simulink model "wlan_mac_dcf_hw"  (Simulink 7.7)
settings: Solver=ode45  StartTime=0.0  StopTime=2e4  RelTol=1e-3
PostLoadFcn:
  | wlan_mac_hw_init
InitFcn:
  | wlan_mac_hw_init
StartFcn:
  | wlan_mac_hw_init
values from neighbouring files (symbols this model uses):
  NB_CNTR_NAV = ceil(log2(MAX_NAV * 160))    [wlan_mac_hw_init.m]
  ticks_per_usec = 10    [wlan_mac_hw_init.m]
undefined symbols (not defined in the file or in its folder): gcbh, xlBlockLoadCallback, xlGetNormalizedPeriod
libraries: xbsIndex_r4 x552, xbsEDKLib_r4 x1
(part 3 of 5)

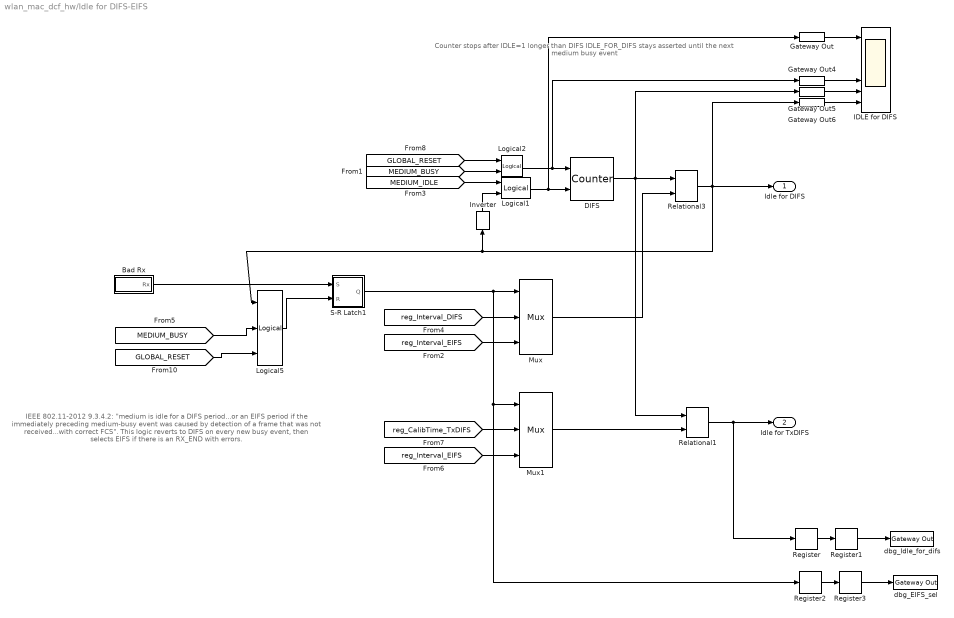
== system wlan_mac_dcf_hw/Idle for DIFS-EIFS ==
  note: IEEE 802.11-2012 9.3.4.2:
      | "medium is idle for a DIFS period...or an EIFS period if the immediately preceding medium-busy
      | event was caused by detection of a frame that was not received...with correct FCS".
      |
      | This logic reverts to DIFS on every new busy event, then
      | selects EIFS if there is an RX_END with errors.
  note: Counter stops after IDLE=1 longer than DIFS
      | IDLE_FOR_DIFS stays asserted until
      | the next medium busy event
  Bad Rx : Subsystem
  DIFS : xbsIndex_r4/Counter  cnt_type=Free Running  cnt_to=inf  operation=Up  start_count=0  cnt_by_val=1  arith_type=Unsigned  n_bits=NB_CNTR_DIFS  bin_pt=0  load_pin=off  rst=on  en=on  explicit_period=off  period=1  dbl_ovrd=off  use_behavioral_HDL=off  implementation=Fabric  block_type=counter
  Gateway Out{,4..6} (4 alike) : xbsIndex_r4/Gateway Out  inherit_from_input=off  hdl_port=off  timing_constraint=None  locs_specified=off  LOCs={}  UseAsDAC=off  DACChannel='1'  block_type=gatewayout
  IDLE for DIFS : Scope  NumInputPorts=7
      settings: YMin=-5~-5~-5~-5~-5~-5~-5  YMax=5~5~5~5~5~5~5  SaveName=ScopeData4
  Inverter : xbsIndex_r4/Inverter  en=off  latency=0  dbl_ovrd=off  block_type=inv
      settings: xl_area=[0 0 0 0 0 0 0]  block_version=VER_STRING_GOES_HERE
  Logical1 : xbsIndex_r4/Logical  logical_function=AND  inputs=2  en=off  latency=0  precision=Full  arith_type=Unsigned  n_bits=16  bin_pt=0  align_bp=on  dbl_ovrd=off  block_type=logical
  Logical2 : xbsIndex_r4/Logical  logical_function=OR  inputs=2  en=off  latency=0  precision=Full  arith_type=Unsigned  n_bits=8  bin_pt=2  align_bp=on  dbl_ovrd=off  block_type=logical
      settings: xl_area=[1 0 0 1 0 0 0]  block_version=VER_STRING_GOES_HERE
  Logical5 : xbsIndex_r4/Logical  logical_function=OR  inputs=3  en=off  latency=0  precision=Full  arith_type=Unsigned  n_bits=16  bin_pt=0  align_bp=on  dbl_ovrd=off  block_type=logical
  Mux : xbsIndex_r4/Mux  inputs=2  en=off  latency=0  precision=Full  arith_type=Unsigned  n_bits=16  bin_pt=14  quantization=Truncate  overflow=Wrap  dbl_ovrd=off  block_type=mux
  Mux1 : xbsIndex_r4/Mux  inputs=2  en=off  latency=0  precision=Full  arith_type=Unsigned  n_bits=16  bin_pt=14  quantization=Truncate  overflow=Wrap  dbl_ovrd=off  block_type=mux
  Register{,1..3} (4 alike) : xbsIndex_r4/Register  init=0  rst=off  en=off  dbl_ovrd=off  block_type=register
  Relational1 : xbsIndex_r4/Relational  mode=a>=b  en=off  latency=0  dbl_ovrd=off  block_type=relational
  Relational3 : xbsIndex_r4/Relational  mode=a>=b  en=off  latency=0  dbl_ovrd=off  block_type=relational
  S-R Latch1 : Subsystem
  dbg_EIFS_sel : xbsIndex_r4/Gateway Out  inherit_from_input=off  hdl_port=on  timing_constraint=None  locs_specified=off  LOCs={}  UseAsDAC=off  DACChannel='1'  block_type=gatewayout
  dbg_Idle_for_difs : xbsIndex_r4/Gateway Out  inherit_from_input=off  hdl_port=on  timing_constraint=None  locs_specified=off  LOCs={}  UseAsDAC=off  DACChannel='1'  block_type=gatewayout
  Idle for DIFS : Outport
  Idle for TxDIFS : Outport  Port=2
  wires:
  Relational3/1 -> Idle for DIFS/1, Inverter/1, Logical5/1, Gateway Out6/1
  Mux/1 -> Relational3/2
  DIFS/1 -> Relational3/1, Relational1/1, Gateway Out5/1
  Logical2/1 -> DIFS/1, Gateway Out4/1
  Logical1/1 -> DIFS/2, Gateway Out/1
  [MEDIUM_IDLE] -> Logical1/1
  [reg_Interval_DIFS] -> Mux/2
  [reg_Interval_EIFS] -> Mux/3
  S-R Latch1/1(Q) -> Mux/1, Mux1/1, Register2/1
  Bad Rx/1(Rx) -> S-R Latch1/1(S)
  Logical5/1 -> S-R Latch1/2(R)
  [MEDIUM_BUSY] -> Logical5/2
  [reg_CalibTime_TxDIFS] -> Mux1/2
  [reg_Interval_EIFS] -> Mux1/3
  Mux1/1 -> Relational1/2
  Relational1/1 -> Idle for TxDIFS/1, Register/1
  Inverter/1 -> Logical1/2
  Gateway Out/1 -> IDLE for DIFS/1
  Gateway Out4/1 -> IDLE for DIFS/5
  Gateway Out5/1 -> IDLE for DIFS/6
  Gateway Out6/1 -> IDLE for DIFS/7
  [GLOBAL_RESET] -> Logical5/3
  [MEDIUM_BUSY] -> Logical2/2
  [GLOBAL_RESET] -> Logical2/1
  Register/1 -> Register1/1
  Register1/1 -> dbg_Idle_for_difs/1
  Register2/1 -> Register3/1
  Register3/1 -> dbg_EIFS_sel/1

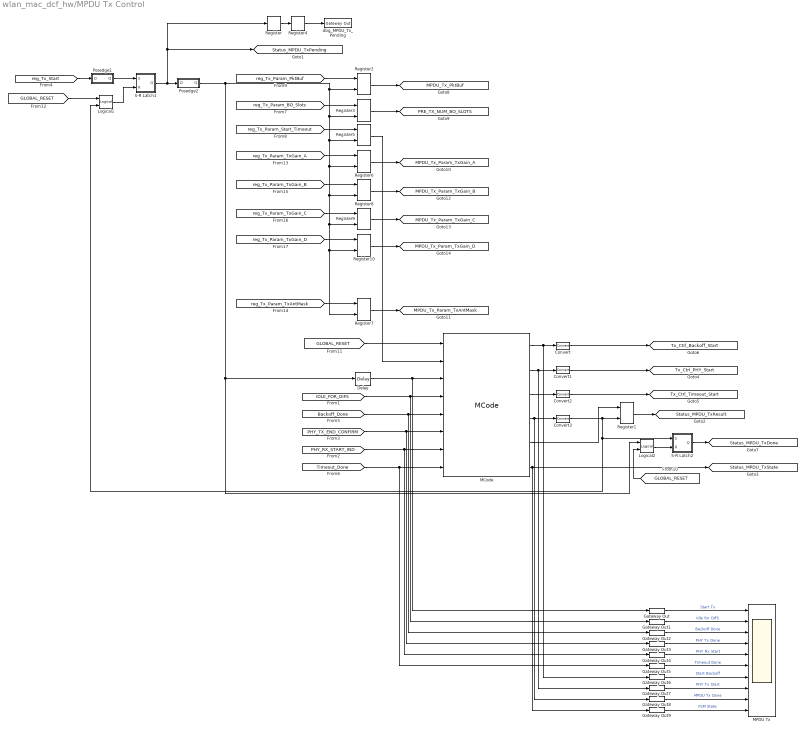
== system wlan_mac_dcf_hw/MPDU Tx Control ==
  Convert{,1..3} (4 alike) : xbsIndex_r4/Convert  gui_display_data_type=Boolean  arith_type=Boolean  n_bits=16  bin_pt=14  float_type=Single  exp_bits=8  fraction_bits=24  quantization=Truncate  overflow=Wrap  en=off  latency=0  dbl_ovrd=off  pipeline=off  block_type=convert
  Delay : xbsIndex_r4/Delay  rst=off  infoeditControl=Selection of Reset will increase slice count due to use of real FFs and instead of SRLs  en=off  latency=1  dbl_ovrd=off  reg_retiming=off  block_type=delay
  Gateway Out{,1..9} (10 alike) : xbsIndex_r4/Gateway Out  inherit_from_input=off  hdl_port=off  timing_constraint=None  locs_specified=off  LOCs={}  UseAsDAC=off  DACChannel='1'  block_type=gatewayout
  Logical1 : xbsIndex_r4/Logical  logical_function=OR  inputs=2  en=off  latency=0  precision=Full  arith_type=Unsigned  n_bits=8  bin_pt=2  align_bp=on  dbl_ovrd=off  block_type=logical
      settings: xl_area=[1 0 0 1 0 0 0]  block_version=VER_STRING_GOES_HERE
  Logical2 : xbsIndex_r4/Logical  logical_function=OR  inputs=2  en=off  latency=0  precision=Full  arith_type=Unsigned  n_bits=8  bin_pt=2  align_bp=on  dbl_ovrd=off  block_type=logical
      settings: xl_area=[1 0 0 1 0 0 0]  block_version=VER_STRING_GOES_HERE
  MCode : xbsIndex_r4/MCode  mfname=mac_tx_ctrl_fsm  explicit_period=on  period=1  inputsTable={'boundInpExpr'=>['','','','','','','',''],'inputs'=>['reset','timeout_req','new_tx','idle_for_difs','backoff_done','phy_tx_done','phy_rx_start','timeout_done']}  outputsTable={'outputs'=>['backoff_start','phy_tx_start','timeout_start','tx_done','tx_result_out','fsm_state_out'],'suppressOut'=>['off','off','off','off','off','off']}  dbl_ovrd=off  enable_stdout=off  enable_debug=off  suppress_output=on  defparams={}  hide_port_list={}  block_type=mcode
  MPDU Tx : Scope  NumInputPorts=10
      settings: YMin=-5~-5~-5~-5~-5~-5~-5~-5~-5~-5  YMax=5~5~5~5~5~5~5~5~5~5
  Posedge1 : Subsystem
  Posedge2 : Subsystem
  Register : xbsIndex_r4/Register  init=0  rst=off  en=off  dbl_ovrd=off  block_type=register
  Register{1..3,5..10} (9 alike) : xbsIndex_r4/Register  init=0  rst=off  en=on  dbl_ovrd=off  block_type=register
  Register4 : xbsIndex_r4/Register  init=0  rst=off  en=off  dbl_ovrd=off  block_type=register
  S-R Latch1 : Subsystem
  S-R Latch2 : Subsystem
  dbg_MPDU_Tx_Pending : xbsIndex_r4/Gateway Out  inherit_from_input=off  hdl_port=on  timing_constraint=None  locs_specified=off  LOCs={}  UseAsDAC=off  DACChannel='1'  block_type=gatewayout
  tag scope: MPDU_Tx_Param_TxAntMask=global, MPDU_Tx_Param_TxGain_A=global, MPDU_Tx_Param_TxGain_B=global, MPDU_Tx_Param_TxGain_C=global, MPDU_Tx_Param_TxGain_D=global, MPDU_Tx_PktBuf=global, PRE_TX_NUM_BO_SLOTS=global, Status_MPDU_TxDone=global, Status_MPDU_TxPending=global, Status_MPDU_TxResult=global, Status_MPDU_TxState=global, Tx_Ctrl_Backoff_Start=global, Tx_Ctrl_PHY_Start=global, Tx_Ctrl_Timeout_Start=global
  wires:
  [reg_Tx_Param_BO_Slots] -> Register3/1
  [reg_Tx_Start] -> Posedge1/1(D)
  Posedge1/1(Q) -> S-R Latch1/1(S)
  S-R Latch1/1(Q) -> Posedge2/1(D), [Status_MPDU_TxPending], Register/1
  Posedge2/1(Q) -> Register3/2, Register5/2, Register6/2, Register8/2, Register9/2, Register7/2, Register10/2, Register2/2, Delay/1, Logical2/1
  Register3/1 -> [PRE_TX_NUM_BO_SLOTS]
  [reg_Tx_Param_PktBuf] -> Register2/1
  Register2/1 -> [MPDU_Tx_PktBuf]
  [reg_Tx_Param_Start_Timeout] -> Register5/1
  Delay/1 -> MCode/3, Gateway Out/1
  Register5/1 -> MCode/2
  [IDLE_FOR_DIFS] -> MCode/4, Gateway Out1/1
  [Backoff_Done] -> MCode/5, Gateway Out2/1
  [PHY_TX_END_CONFIRM] -> MCode/6, Gateway Out3/1
  [PHY_RX_START_IND] -> MCode/7, Gateway Out4/1
  [Timeout_Done] -> MCode/8, Gateway Out5/1
  [GLOBAL_RESET] -> MCode/1
  Logical1/1 -> S-R Latch1/2(R)
  [GLOBAL_RESET] -> Logical1/1
  MCode/4 -> Convert3/1, Gateway Out8/1
  MCode/2 -> Convert1/1, Gateway Out7/1
  MCode/3 -> Convert2/1
  MCode/1 -> Convert/1, Gateway Out6/1
  MCode/5 -> Register1/1
  Register1/1 -> [Status_MPDU_TxResult]
  MCode/6 -> [Status_MPDU_TxState], Gateway Out9/1
  S-R Latch2/1(Q) -> [Status_MPDU_TxDone]
  Convert/1 -> [Tx_Ctrl_Backoff_Start]
  Convert1/1 -> [Tx_Ctrl_PHY_Start]
  Convert2/1 -> [Tx_Ctrl_Timeout_Start]
  Convert3/1 -> Register1/2, S-R Latch2/1(S), Logical1/2
  Logical2/1 -> S-R Latch2/2(R)
  [GLOBAL_RESET] -> Logical2/2
  Gateway Out/1 -> MPDU Tx/1  "Start Tx"
  Gateway Out1/1 -> MPDU Tx/2  "Idle for DIFS"
  Gateway Out2/1 -> MPDU Tx/3  "Backoff Done"
  Gateway Out3/1 -> MPDU Tx/4  "PHY Tx Done"
  Gateway Out4/1 -> MPDU Tx/5  "PHY Rx Start"
  Gateway Out5/1 -> MPDU Tx/6  "Timeout Done"
  Gateway Out6/1 -> MPDU Tx/7  "Start Backoff"
  Gateway Out7/1 -> MPDU Tx/8  "PHY Tx Start"
  Gateway Out8/1 -> MPDU Tx/9  "MPDU Tx Done"
  Gateway Out9/1 -> MPDU Tx/10  "FSM State"
  Register/1 -> Register4/1
  Register4/1 -> dbg_MPDU_Tx_Pending/1
  [reg_Tx_Param_TxGain_A] -> Register6/1
  Register6/1 -> [MPDU_Tx_Param_TxGain_A]
  [reg_Tx_Param_TxAntMask] -> Register7/1
  Register7/1 -> [MPDU_Tx_Param_TxAntMask]
  [reg_Tx_Param_TxGain_B] -> Register8/1
  [reg_Tx_Param_TxGain_C] -> Register9/1
  [reg_Tx_Param_TxGain_D] -> Register10/1
  Register8/1 -> [MPDU_Tx_Param_TxGain_B]
  Register9/1 -> [MPDU_Tx_Param_TxGain_C]
  Register10/1 -> [MPDU_Tx_Param_TxGain_D]

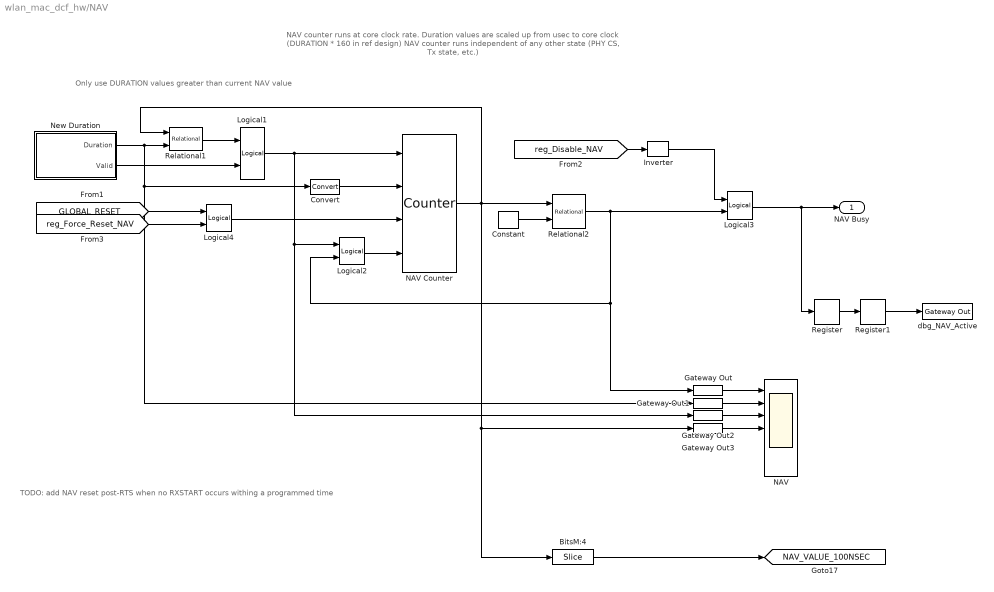
== system wlan_mac_dcf_hw/NAV ==
  note: NAV counter runs at core clock rate. Duration
      | values are scaled up from usec to core clock
      | (DURATION * 160 in ref design)
      |
      | NAV counter runs independent of any
      | other state (PHY CS, Tx state, etc.)
  note: Only use DURATION values greater
      | than current NAV value
  note: TODO: add NAV reset post-RTS when no RXSTART occurs
      | withing a programmed time
  BitsM:4 : xbsIndex_r4/Slice  nbits=NB_CNTR_NAV-4  boolean_output=off  mode=Upper Bit Location + Width  bit1=0  base1=MSB of Input  bit0=0  base0=LSB of Input  dbl_ovrd=off  block_type=slice
  Constant : xbsIndex_r4/Constant  const=0  gui_display_data_type=Fixed-point  arith_type=Unsigned  n_bits=1  bin_pt=0  preci_type=Single  exp_width=8  frac_width=24  explicit_period=off  period=1  equ=P=C  opselect=C  inp2=PCIN>>17  opr=+  inp1=P  carry=CIN  dbl_ovrd=off  block_type=constant
  Convert : xbsIndex_r4/Convert  gui_display_data_type=Fixed-point  arith_type=Unsigned  n_bits=NB_CNTR_NAV  bin_pt=0  float_type=Single  exp_bits=8  fraction_bits=24  quantization=Truncate  overflow=Wrap  en=off  latency=0  dbl_ovrd=off  pipeline=off  block_type=convert
  Gateway Out{,1..3} (4 alike) : xbsIndex_r4/Gateway Out  inherit_from_input=off  hdl_port=off  timing_constraint=None  locs_specified=off  LOCs={}  UseAsDAC=off  DACChannel='1'  block_type=gatewayout
  Inverter : xbsIndex_r4/Inverter  en=off  latency=0  dbl_ovrd=off  block_type=inv
      settings: xl_area=[0 0 0 0 0 0 0]  block_version=VER_STRING_GOES_HERE
  Logical1 : xbsIndex_r4/Logical  logical_function=AND  inputs=2  en=off  latency=0  precision=Full  arith_type=Unsigned  n_bits=16  bin_pt=0  align_bp=on  dbl_ovrd=off  block_type=logical
  Logical2 : xbsIndex_r4/Logical  logical_function=OR  inputs=2  en=off  latency=0  precision=Full  arith_type=Unsigned  n_bits=16  bin_pt=0  align_bp=on  dbl_ovrd=off  block_type=logical
  Logical3 : xbsIndex_r4/Logical  logical_function=AND  inputs=2  en=off  latency=0  precision=Full  arith_type=Unsigned  n_bits=16  bin_pt=0  align_bp=on  dbl_ovrd=off  block_type=logical
  Logical4 : xbsIndex_r4/Logical  logical_function=OR  inputs=2  en=off  latency=0  precision=Full  arith_type=Unsigned  n_bits=16  bin_pt=0  align_bp=on  dbl_ovrd=off  block_type=logical
  NAV : Scope  NumInputPorts=7
      settings: YMin=-5~-5~-5~-5~-5~-5~-5  YMax=5~5~5~5~5~5~5  SaveName=ScopeData3
  NAV Counter : xbsIndex_r4/Counter  cnt_type=Free Running  cnt_to=Inf  operation=Down  start_count=0  cnt_by_val=1  arith_type=Unsigned  n_bits=NB_CNTR_NAV  bin_pt=0  load_pin=on  rst=on  en=on  explicit_period=on  period=1  dbl_ovrd=off  use_behavioral_HDL=off  implementation=Fabric  block_type=counter
  New Duration : Subsystem
  Register : xbsIndex_r4/Register  init=0  rst=off  en=off  dbl_ovrd=off  block_type=register
  Register1 : xbsIndex_r4/Register  init=0  rst=off  en=off  dbl_ovrd=off  block_type=register
  Relational1 : xbsIndex_r4/Relational  mode=a<b  en=off  latency=0  dbl_ovrd=off  block_type=relational
  Relational2 : xbsIndex_r4/Relational  mode=a>b  en=off  latency=0  dbl_ovrd=off  block_type=relational
  dbg_NAV_Active : xbsIndex_r4/Gateway Out  inherit_from_input=off  hdl_port=on  timing_constraint=None  locs_specified=off  LOCs={}  UseAsDAC=off  DACChannel='1'  block_type=gatewayout
  NAV Busy : Outport
  tag scope: NAV_VALUE_100NSEC=global
  wires:
  Logical1/1 -> NAV Counter/1, Logical2/1, Gateway Out2/1
  New Duration/2(Valid) -> Logical1/2
  NAV Counter/1 -> Relational2/1, Relational1/1, Gateway Out3/1, BitsM:4/1
  Logical4/1 -> NAV Counter/3
  Constant/1 -> Relational2/2
  Relational2/1 -> Gateway Out/1, Logical2/2, Logical3/2
  New Duration/1(Duration) -> Relational1/2, Convert/1, Gateway Out1/1
  Relational1/1 -> Logical1/1
  Convert/1 -> NAV Counter/2
  Gateway Out/1 -> NAV/1
  Gateway Out1/1 -> NAV/2
  Gateway Out2/1 -> NAV/3
  Gateway Out3/1 -> NAV/4
  Logical2/1 -> NAV Counter/4
  Logical3/1 -> NAV Busy/1, Register/1
  [reg_Disable_NAV] -> Inverter/1
  Inverter/1 -> Logical3/1
  Register/1 -> Register1/1
  Register1/1 -> dbg_NAV_Active/1
  BitsM:4/1 -> [NAV_VALUE_100NSEC]
  [GLOBAL_RESET] -> Logical4/1
  [reg_Force_Reset_NAV] -> Logical4/2

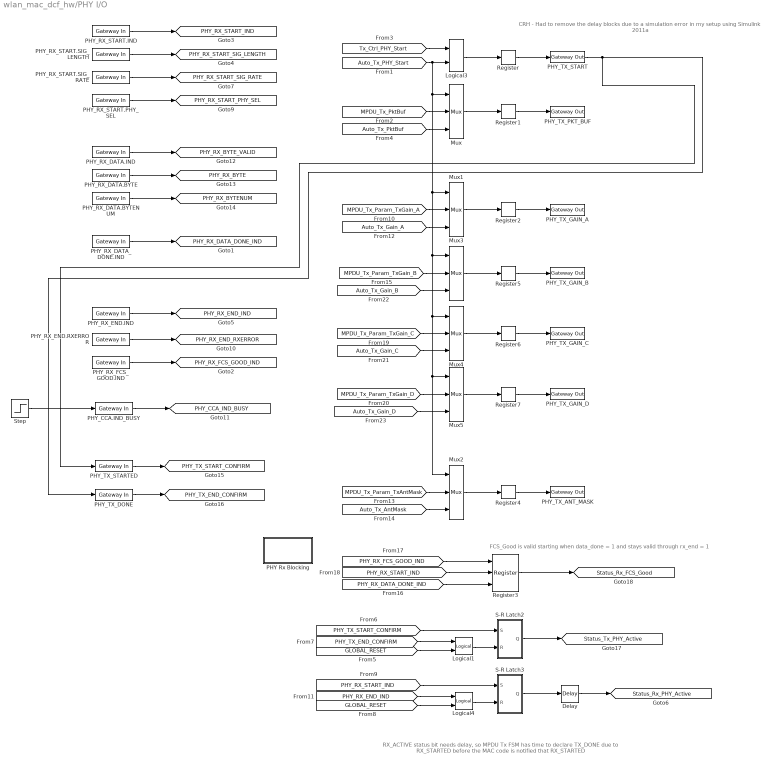
== system wlan_mac_dcf_hw/PHY I/O ==
  note: FCS_Good is valid starting when
      | data_done = 1 and stays valid through
      | rx_end = 1
  note: RX_ACTIVE status bit needs delay, so MPDU Tx FSM has time to declare TX_DONE
      |   due to RX_STARTED before the MAC code is notified that RX_STARTED
  note: CRH - Had to remove
      | the delay blocks due
      | to a simulation error
      | in my setup using
      | Simulink 2011a
  Delay : xbsIndex_r4/Delay  rst=off  infoeditControl=Selection of Reset will increase slice count due to use of real FFs and instead of SRLs  en=off  latency=3  dbl_ovrd=off  reg_retiming=off  block_type=delay
  Logical1 : xbsIndex_r4/Logical  logical_function=OR  inputs=2  en=off  latency=0  precision=Full  arith_type=Unsigned  n_bits=8  bin_pt=2  align_bp=on  dbl_ovrd=off  block_type=logical
      settings: xl_area=[1 0 0 1 0 0 0]  block_version=VER_STRING_GOES_HERE
  Logical3 : xbsIndex_r4/Logical  logical_function=OR  inputs=2  en=off  latency=0  precision=Full  arith_type=Unsigned  n_bits=16  bin_pt=0  align_bp=on  dbl_ovrd=off  block_type=logical
  Logical4 : xbsIndex_r4/Logical  logical_function=OR  inputs=2  en=off  latency=0  precision=Full  arith_type=Unsigned  n_bits=8  bin_pt=2  align_bp=on  dbl_ovrd=off  block_type=logical
      settings: xl_area=[1 0 0 1 0 0 0]  block_version=VER_STRING_GOES_HERE
  Mux{,1..5} (6 alike) : xbsIndex_r4/Mux  inputs=2  en=off  latency=0  precision=Full  arith_type=Unsigned  n_bits=16  bin_pt=14  quantization=Truncate  overflow=Wrap  dbl_ovrd=off  block_type=mux
  PHY Rx Blocking : Subsystem
  PHY_CCA.IND_BUSY : xbsIndex_r4/Gateway In  gui_display_data_type=Boolean  arith_type=Boolean  n_bits=16  bin_pt=14  preci_type=Single  exp_width=8  frac_width=24  quantization="Round  (unbiased: +/- Inf)"  overflow=Saturate  period=1  dbl_ovrd=off  timing_constraint=None  locs_specified=off  LOCs={}  UseAsADC=off  ADCChannel='1'  inherit_from_input=off  hdl_port=on  block_type=gatewayin
  PHY_RX_DATA.BYTE : xbsIndex_r4/Gateway In  gui_display_data_type=Fixed-point  arith_type=Unsigned  n_bits=8  bin_pt=0  preci_type=Single  exp_width=8  frac_width=24  quantization="Round  (unbiased: +/- Inf)"  overflow=Saturate  period=1  dbl_ovrd=off  timing_constraint=None  locs_specified=off  LOCs={}  UseAsADC=off  ADCChannel='1'  inherit_from_input=off  hdl_port=on  block_type=gatewayin
  PHY_RX_DATA.BYTENUM : xbsIndex_r4/Gateway In  gui_display_data_type=Fixed-point  arith_type=Unsigned  n_bits=14  bin_pt=0  preci_type=Single  exp_width=8  frac_width=24  quantization="Round  (unbiased: +/- Inf)"  overflow=Saturate  period=1  dbl_ovrd=off  timing_constraint=None  locs_specified=off  LOCs={}  UseAsADC=off  ADCChannel='1'  inherit_from_input=off  hdl_port=on  block_type=gatewayin
  PHY_RX_DATA.IND : xbsIndex_r4/Gateway In  gui_display_data_type=Boolean  arith_type=Boolean  n_bits=16  bin_pt=14  preci_type=Single  exp_width=8  frac_width=24  quantization="Round  (unbiased: +/- Inf)"  overflow=Saturate  period=1  dbl_ovrd=off  timing_constraint=None  locs_specified=off  LOCs={}  UseAsADC=off  ADCChannel='1'  inherit_from_input=off  hdl_port=on  block_type=gatewayin
  PHY_RX_DATA_DONE.IND : xbsIndex_r4/Gateway In  gui_display_data_type=Boolean  arith_type=Boolean  n_bits=1  bin_pt=0  preci_type=Single  exp_width=8  frac_width=24  quantization="Round  (unbiased: +/- Inf)"  overflow=Saturate  period=1  dbl_ovrd=off  timing_constraint=None  locs_specified=off  LOCs={}  UseAsADC=off  ADCChannel='1'  inherit_from_input=off  hdl_port=on  block_type=gatewayin
  PHY_RX_END.IND : xbsIndex_r4/Gateway In  gui_display_data_type=Boolean  arith_type=Boolean  n_bits=16  bin_pt=14  preci_type=Single  exp_width=8  frac_width=24  quantization="Round  (unbiased: +/- Inf)"  overflow=Saturate  period=1  dbl_ovrd=off  timing_constraint=None  locs_specified=off  LOCs={}  UseAsADC=off  ADCChannel='1'  inherit_from_input=off  hdl_port=on  block_type=gatewayin
  PHY_RX_END.RXERROR : xbsIndex_r4/Gateway In  gui_display_data_type=Fixed-point  arith_type=Unsigned  n_bits=2  bin_pt=0  preci_type=Single  exp_width=8  frac_width=24  quantization="Round  (unbiased: +/- Inf)"  overflow=Saturate  period=1  dbl_ovrd=off  timing_constraint=None  locs_specified=off  LOCs={}  UseAsADC=off  ADCChannel='1'  inherit_from_input=off  hdl_port=on  block_type=gatewayin
  PHY_RX_FCS_GOOD.IND : xbsIndex_r4/Gateway In  gui_display_data_type=Boolean  arith_type=Boolean  n_bits=1  bin_pt=0  preci_type=Single  exp_width=8  frac_width=24  quantization="Round  (unbiased: +/- Inf)"  overflow=Saturate  period=1  dbl_ovrd=off  timing_constraint=None  locs_specified=off  LOCs={}  UseAsADC=off  ADCChannel='1'  inherit_from_input=off  hdl_port=on  block_type=gatewayin
  PHY_RX_START.IND : xbsIndex_r4/Gateway In  gui_display_data_type=Boolean  arith_type=Boolean  n_bits=16  bin_pt=14  preci_type=Single  exp_width=8  frac_width=24  quantization="Round  (unbiased: +/- Inf)"  overflow=Saturate  period=1  dbl_ovrd=off  timing_constraint=None  locs_specified=off  LOCs={}  UseAsADC=off  ADCChannel='1'  inherit_from_input=off  hdl_port=on  block_type=gatewayin
  PHY_RX_START.PHY_SEL : xbsIndex_r4/Gateway In  gui_display_data_type=Boolean  arith_type=Boolean  n_bits=16  bin_pt=14  preci_type=Single  exp_width=8  frac_width=24  quantization="Round  (unbiased: +/- Inf)"  overflow=Saturate  period=1  dbl_ovrd=off  timing_constraint=None  locs_specified=off  LOCs={}  UseAsADC=off  ADCChannel='1'  inherit_from_input=off  hdl_port=on  block_type=gatewayin
  PHY_RX_START.SIG_LENGTH : xbsIndex_r4/Gateway In  gui_display_data_type=Fixed-point  arith_type=Unsigned  n_bits=12  bin_pt=0  preci_type=Single  exp_width=8  frac_width=24  quantization="Round  (unbiased: +/- Inf)"  overflow=Saturate  period=1  dbl_ovrd=off  timing_constraint=None  locs_specified=off  LOCs={}  UseAsADC=off  ADCChannel='1'  inherit_from_input=off  hdl_port=on  block_type=gatewayin
  PHY_RX_START.SIG_RATE : xbsIndex_r4/Gateway In  gui_display_data_type=Fixed-point  arith_type=Unsigned  n_bits=4  bin_pt=0  preci_type=Single  exp_width=8  frac_width=24  quantization="Round  (unbiased: +/- Inf)"  overflow=Saturate  period=1  dbl_ovrd=off  timing_constraint=None  locs_specified=off  LOCs={}  UseAsADC=off  ADCChannel='1'  inherit_from_input=off  hdl_port=on  block_type=gatewayin
  PHY_TX_ANT_MASK : xbsIndex_r4/Gateway Out  inherit_from_input=off  hdl_port=on  timing_constraint=None  locs_specified=off  LOCs={}  UseAsDAC=off  DACChannel='1'  block_type=gatewayout
  PHY_TX_DONE : xbsIndex_r4/Gateway In  gui_display_data_type=Boolean  arith_type=Boolean  n_bits=16  bin_pt=14  preci_type=Single  exp_width=8  frac_width=24  quantization="Round  (unbiased: +/- Inf)"  overflow=Saturate  period=1  dbl_ovrd=off  timing_constraint=None  locs_specified=off  LOCs={}  UseAsADC=off  ADCChannel='1'  inherit_from_input=off  hdl_port=on  block_type=gatewayin
  PHY_TX_GAIN_A : xbsIndex_r4/Gateway Out  inherit_from_input=off  hdl_port=on  timing_constraint=None  locs_specified=off  LOCs={}  UseAsDAC=off  DACChannel='1'  block_type=gatewayout
  PHY_TX_GAIN_B : xbsIndex_r4/Gateway Out  inherit_from_input=off  hdl_port=on  timing_constraint=None  locs_specified=off  LOCs={}  UseAsDAC=off  DACChannel='1'  block_type=gatewayout
  PHY_TX_GAIN_C : xbsIndex_r4/Gateway Out  inherit_from_input=off  hdl_port=on  timing_constraint=None  locs_specified=off  LOCs={}  UseAsDAC=off  DACChannel='1'  block_type=gatewayout
  PHY_TX_GAIN_D : xbsIndex_r4/Gateway Out  inherit_from_input=off  hdl_port=on  timing_constraint=None  locs_specified=off  LOCs={}  UseAsDAC=off  DACChannel='1'  block_type=gatewayout
  PHY_TX_PKT_BUF : xbsIndex_r4/Gateway Out  inherit_from_input=off  hdl_port=on  timing_constraint=None  locs_specified=off  LOCs={}  UseAsDAC=off  DACChannel='1'  block_type=gatewayout
  PHY_TX_START : xbsIndex_r4/Gateway Out  inherit_from_input=off  hdl_port=on  timing_constraint=None  locs_specified=off  LOCs={}  UseAsDAC=off  DACChannel='1'  block_type=gatewayout
  PHY_TX_STARTED : xbsIndex_r4/Gateway In  gui_display_data_type=Boolean  arith_type=Boolean  n_bits=16  bin_pt=14  preci_type=Single  exp_width=8  frac_width=24  quantization="Round  (unbiased: +/- Inf)"  overflow=Saturate  period=1  dbl_ovrd=off  timing_constraint=None  locs_specified=off  LOCs={}  UseAsADC=off  ADCChannel='1'  inherit_from_input=off  hdl_port=on  block_type=gatewayin
  Register{,1..2,4..7} (7 alike) : xbsIndex_r4/Register  init=0  rst=off  en=off  dbl_ovrd=off  block_type=register
  Register3 : xbsIndex_r4/Register  init=0  rst=on  en=on  dbl_ovrd=off  block_type=register
  S-R Latch2 : Subsystem
  S-R Latch3 : Subsystem
  Step : Step  Time=6e3  Before=1  After=0  SampleTime=1
  tag scope: PHY_CCA_IND_BUSY=global, PHY_RX_BYTE=global, PHY_RX_BYTENUM=global, PHY_RX_BYTE_VALID=global, PHY_RX_DATA_DONE_IND=global, PHY_RX_END_IND=global, PHY_RX_END_RXERROR=global, PHY_RX_FCS_GOOD_IND=global, PHY_RX_START_IND=global, PHY_RX_START_PHY_SEL=global, PHY_RX_START_SIG_LENGTH=global, PHY_RX_START_SIG_RATE=global, PHY_TX_END_CONFIRM=global, PHY_TX_START_CONFIRM=global, Status_Rx_FCS_Good=global, Status_Rx_PHY_Active=global, Status_Tx_PHY_Active=global
  wires:
  PHY_RX_DATA_DONE.IND/1 -> [PHY_RX_DATA_DONE_IND]
  PHY_RX_FCS_GOOD.IND/1 -> [PHY_RX_FCS_GOOD_IND]
  PHY_RX_START.IND/1 -> [PHY_RX_START_IND]
  PHY_RX_START.SIG_LENGTH/1 -> [PHY_RX_START_SIG_LENGTH]
  PHY_RX_END.IND/1 -> [PHY_RX_END_IND]
  PHY_RX_END.RXERROR/1 -> [PHY_RX_END_RXERROR]
  PHY_CCA.IND_BUSY/1 -> [PHY_CCA_IND_BUSY]
  PHY_RX_DATA.IND/1 -> [PHY_RX_BYTE_VALID]
  PHY_RX_DATA.BYTE/1 -> [PHY_RX_BYTE]
  PHY_RX_DATA.BYTENUM/1 -> [PHY_RX_BYTENUM]
  PHY_TX_STARTED/1 -> [PHY_TX_START_CONFIRM]
  PHY_TX_DONE/1 -> [PHY_TX_END_CONFIRM]
  Logical3/1 -> Register/1
  [Tx_Ctrl_PHY_Start] -> Logical3/1
  [Auto_Tx_PHY_Start] -> Logical3/2, Mux/1, Mux1/1, Mux3/1, Mux4/1, Mux2/1, Mux5/1
  Mux/1 -> Register1/1
  [MPDU_Tx_PktBuf] -> Mux/2
  [Auto_Tx_PktBuf] -> Mux/3
  Register/1 -> PHY_TX_START/1
  Register1/1 -> PHY_TX_PKT_BUF/1
  [PHY_TX_START_CONFIRM] -> S-R Latch2/1(S)
  Logical1/1 -> S-R Latch2/2(R)
  [PHY_TX_END_CONFIRM] -> Logical1/1
  [GLOBAL_RESET] -> Logical1/2
  S-R Latch2/1(Q) -> [Status_Tx_PHY_Active]
  [PHY_RX_START_IND] -> S-R Latch3/1(S)
  Logical4/1 -> S-R Latch3/2(R)
  [PHY_RX_END_IND] -> Logical4/1
  [GLOBAL_RESET] -> Logical4/2
  S-R Latch3/1(Q) -> Delay/1
  PHY_RX_START.SIG_RATE/1 -> [PHY_RX_START_SIG_RATE]
  PHY_RX_START.PHY_SEL/1 -> [PHY_RX_START_PHY_SEL]
  [PHY_RX_FCS_GOOD_IND] -> Register3/1
  Register3/1 -> [Status_Rx_FCS_Good]
  [PHY_RX_DATA_DONE_IND] -> Register3/3
  [PHY_RX_START_IND] -> Register3/2
  Delay/1 -> [Status_Rx_PHY_Active]
  PHY_TX_START/1 -> PHY_TX_DONE/1, PHY_TX_STARTED/1
  Step/1 -> PHY_CCA.IND_BUSY/1
  Mux1/1 -> Register2/1
  [MPDU_Tx_Param_TxGain_A] -> Mux1/2
  [Auto_Tx_Gain_A] -> Mux1/3
  Register2/1 -> PHY_TX_GAIN_A/1
  Mux2/1 -> Register4/1
  Register4/1 -> PHY_TX_ANT_MASK/1
  [MPDU_Tx_Param_TxAntMask] -> Mux2/2
  [Auto_Tx_AntMask] -> Mux2/3
  Mux3/1 -> Register5/1
  Register5/1 -> PHY_TX_GAIN_B/1
  Mux4/1 -> Register6/1
  Register6/1 -> PHY_TX_GAIN_C/1
  Mux5/1 -> Register7/1
  Register7/1 -> PHY_TX_GAIN_D/1
  [MPDU_Tx_Param_TxGain_B] -> Mux3/2
  [MPDU_Tx_Param_TxGain_C] -> Mux4/2
  [MPDU_Tx_Param_TxGain_D] -> Mux5/2
  [Auto_Tx_Gain_B] -> Mux3/3
  [Auto_Tx_Gain_C] -> Mux4/3
  [Auto_Tx_Gain_D] -> Mux5/3
